simulink model "counter"  (R2018b)
settings: Solver=VariableStepAuto  StartTime=0.0  StopTime=10.0  RelTol=1e-3
libraries: simulink x3
settings Model: Creator=Hiro  LastModifiedBy=Hiro

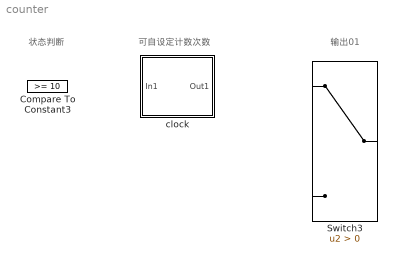
== system counter ==
  note: 可自设定计数次数
  note: 输出01
  note: 状态判断
  Compare To Constant3 : simulink/Logic and Bit Operations/Compare To Constant  relop=>=  const=10  OutDataTypeStr=boolean
  Switch3 : Switch  Criteria=u2 > Threshold  OutDataTypeStr=uint16
  clock : Subsystem

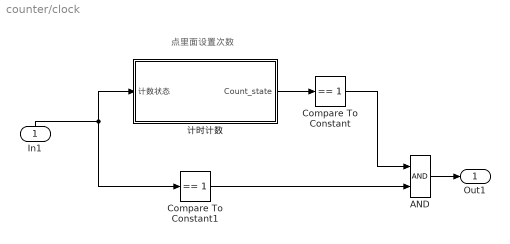
== system counter/clock ==
  note: 点里面设置次数
  In1 : Inport
  AND : Logic  IconShape=distinctive  AllPortsSameDT=off  OutDataTypeStr=boolean
  Compare To Constant : simulink/Logic and Bit Operations/Compare To Constant  relop===  const=1  OutDataTypeStr=boolean
  Compare To Constant1 : simulink/Logic and Bit Operations/Compare To Constant  relop===  const=1  OutDataTypeStr=boolean
  计时计数 : Subsystem  Description=计数模块，当有输入信号有跳变的时候会触发使计数值清零  TreatAsAtomicUnit=on
  Out1 : Outport
  wires:
  Compare To Constant1/1 -> AND/2
  Compare To Constant/1 -> AND/1
  计时计数/1(Count_state) -> Compare To Constant/1
  In1/1 -> 计时计数/1(计数状态), Compare To Constant1/1
  AND/1 -> Out1/1

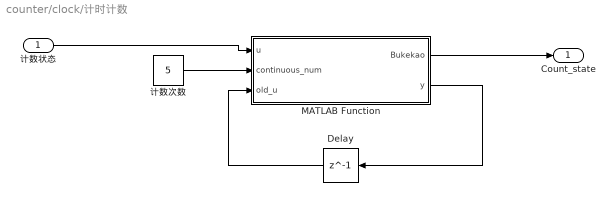
== system counter/clock/计时计数 ==
  计数状态 : Inport
  Delay : Delay  DelayLength=1
  MATLAB Function : MATLAB Function  TreatAsAtomicUnit=on
  计数次数 : Constant  Value=5  SampleTime=-1
  Count_state : Outport
  wires:
  MATLAB Function/2(y) -> Delay/1
  Delay/1 -> MATLAB Function/3(old_u)
  MATLAB Function/1(Bukekao) -> Count_state/1
  计数状态/1 -> MATLAB Function/1(u)
  计数次数/1 -> MATLAB Function/2(continuous_num)

== matlab function counter/clock/计时计数/MATLAB Function ==
  data: Bukekao output; u input; y output; continuous_num input; old_u input
function [Bukekao,y] = fcn(u,continuous_num,old_u)
%
%
%出现踏板不可靠
if(u==1)
    y = 1+old_u;        %输出的不可靠次数y = 累计次数 + 1；
else
    y=0;                %输出可靠后清除不可靠信号
end
if(y>continuous_num)    %当不可靠次数y > 设定的阈值次数
    Bukekao=1;          %不可靠输出 1 
else
    Bukekao=0;          %否则不可靠输出 0
end
if(y>100)
    y = 100;
end
